simulink model "Chapter_9_Section_3_3"  (R2026a)
settings: Solver=FixedStepAuto  FixedStep=0.02  EnableMultiTasking=on
libraries: arduinolib x2, simulink x1
settings Model: SILPILModeSetting=veronly  ExtModeTrigDuration=2  Creator=ASUS  LastModifiedBy=ASUS
settings HardwareCC: ProdBitPerInt=16.0  ProdBitPerPointer=16.0  ProdBitPerSizeT=16.0  ProdBitPerPtrDiffT=16.0  ProdWordSize=8.0  ProdHWDeviceType=Atmel->AVR  UseEmbeddedCoderFeatures=off
settings RTWCC: SystemTargetFile=ert.tlc  HardwareBoard=Arduino Mega 2560  TLCOptions=-aInlineSetEventsForThisBaseRateFcn=TLC_FALSE -aSuppressMultiTaskScheduler=TLC_FALSE -aRateBasedStepFcn=1  Toolchain=Arduino AVR  BuildConfiguration=Faster Runs  Description=Embedded Coder
settings ERTTargetCC: ExtModeTransport=3.0  ExtModeAutomaticAllocSize=off  ExtModeStaticAllocSize=2048.0  SupportContinuousTime=on  SupportNonInlinedSFcns=on  SupportVariableSizeSignals=on

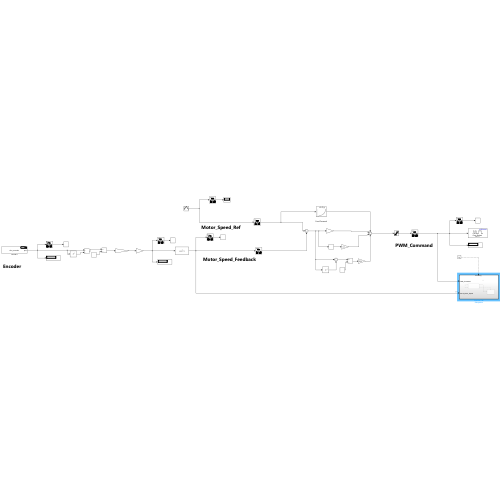
[thumbnail: Simulink's stored preview of the top-level diagram]
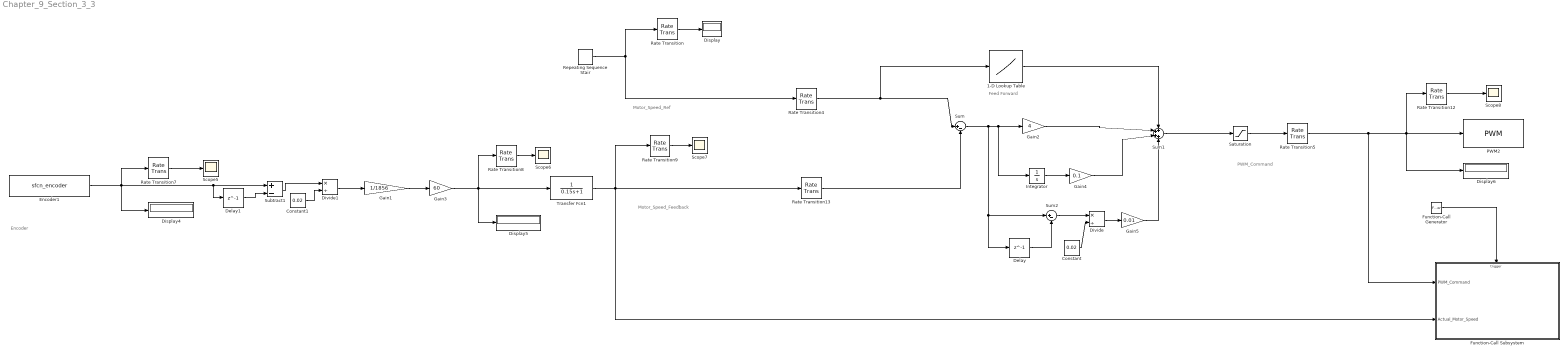
== system Chapter_9_Section_3_3 ==
  note: Feed Forward
  note: Motor_Speed_Ref
  note: Motor_Speed_Feedback
  note: PWM_Command
  note: Encoder
  1-D Lookup Table : Lookup_n-D  NumberOfTableDimensions=1  BreakpointsForDimension1=[78.1 185.9 260.2 305.1 331.5 351 363.3 374.1 382.7 394.4]  Table=[25.5 50.1 76.5 102 127.5 153 178.5 204 229.5 255]  InternalRulePriority=Speed  RndMeth=Simplest
  Constant : Constant  Value=0.02
  Constant1 : Constant  Value=0.02
  Delay : Delay  DelayLength=1  InitialCondition=0
  Delay1 : Delay  DelayLength=1  InitialCondition=0
  Display{,4..6} (4 alike) : Display
  Divide : Product  Inputs=*/
  Divide1 : Product  Inputs=*/
  Encoder1 : S-Function  InitFcn=try, set_param(gcb,'FunctionName','sfcn_encoder'), end  FunctionName=sfcn_encoder  Parameters=uint8(0),uint8(2),uint8(3)  SFunctionModules=sfcn_encoder_wrapper.c  SFunctionDeploymentMode=off  EnableBusSupport=off  mask(S-Function Builder){}
      mask init:
      | val = [[.9  0.75 0.75 1 1 .9 .9 1]',[1 1 0.75 0.75 .9 .9 1 .9]'];try , sys = get_param(gcb,'SfunBuilderFcnName');if isempty(sys), sys = get_param(gcb,'FunctionName'); end,catch, sys = get_param(gcb,'FunctionName'); end
      settings: CopyFcn=set_param(gcbh,'LinkStatus','none')  PreSaveFcn=try, set_param(gcb,'FunctionName','sfcn_encoder'), end  OpenFcn=sfunctionwizard(gcbh)
      mask Display:
      | plot(val(:,1),val(:,2))
      | disp(sys)
      | port_label('output',1,sprintf('%s', 'pos'),'interpreter','tex')
  Function-Call Generator : FunctionCallGenerator  SampleTime=0.1
  Function-Call Subsystem : Subsystem  TreatAsAtomicUnit=on
  Gain1 : Gain  Gain=1/1856
  Gain2 : Gain  Gain=4
  Gain3 : Gain  Gain=60
  Gain4 : Gain  Gain=0.1
  Gain5 : Gain  Gain=0.01
  Integrator : Integrator
  PWM2 : arduinolib/PWM  pinNumber=5  frequencyType=Default  desiredFrequency=490.2  achievableFrequency=490.1961
  Rate Transition{,4..5,7..9,12..13} (8 alike) : RateTransition
  Repeating Sequence Stair : simulink/Sources/Repeating Sequence Stair  OutValues=[110:200 199:-1:110]  tsamp=0.2  OutMin=[]  OutMax=[]  OutDataTypeStr=double  OutputDataTypeScalingMode=double  OutDataType=fixdt(0,8)  ConRadixGroup=Best Precision: Vector-wise  OutScaling=2^-12
  Saturation : Saturate  UpperLimit=255  LowerLimit=0
  Scope{5..8} (4 alike) : Scope
      Scope5 settings: ActiveDisplayYMinimum=-22.407200582277603  ActiveDisplayYMaximum=19.171363005949797  DataLoggingVariableName=ScopeData5
      Scope6 settings: ActiveDisplayYMinimum=-22.407200582277603  ActiveDisplayYMaximum=19.171363005949797  DataLoggingVariableName=ScopeData6
      Scope7 settings: ActiveDisplayYMinimum=-22.407200582277603  ActiveDisplayYMaximum=19.171363005949797  DataLoggingVariableName=ScopeData7
      Scope8 settings: ActiveDisplayYMinimum=-11.899191623313698  ActiveDisplayYMaximum=179.03299178469436  DataLoggingVariableName=ScopeData8
  Subtract1 : Sum  Inputs=+-
  Sum : Sum  Inputs=|+-
  Sum1 : Sum  Inputs=++++
  Sum2 : Sum  Inputs=|+-
  Transfer Fcn1 : TransferFcn  Denominator=[0.15 1]
  wires:
  Gain4/1 -> Sum1/3
  Divide/1 -> Gain5/1
  Gain5/1 -> Sum1/4
  Delay/1 -> Sum2/2
  Constant/1 -> Divide/2
  Sum1/1 -> Saturation/1
  Sum2/1 -> Divide/1
  Integrator/1 -> Gain4/1
  1-D Lookup Table/1 -> Sum1/1
  Rate Transition13/1 -> Sum/2
  Rate Transition4/1 -> 1-D Lookup Table/1, Sum/1
  Gain2/1 -> Sum1/2
  Sum/1 -> Sum2/1, Delay/1, Integrator/1, Gain2/1
  Saturation/1 -> Rate Transition5/1
  Rate Transition8/1 -> Scope6/1
  Delay1/1 -> Subtract1/2
  Rate Transition7/1 -> Scope5/1
  Subtract1/1 -> Divide1/1
  Transfer Fcn1/1 -> Function-Call Subsystem/2(Actual_Motor_Speed), Rate Transition13/1, Rate Transition9/1
  Rate Transition9/1 -> Scope7/1
  Gain1/1 -> Gain3/1
  Divide1/1 -> Gain1/1
  Constant1/1 -> Divide1/2
  Encoder1/1 -> Subtract1/1, Delay1/1, Rate Transition7/1, Display4/1
  Gain3/1 -> Transfer Fcn1/1, Display5/1, Rate Transition8/1
  Repeating Sequence Stair/1 -> Rate Transition4/1, Rate Transition/1
  Rate Transition/1 -> Display/1
  Rate Transition12/1 -> Scope8/1
  Rate Transition5/1 -> Function-Call Subsystem/1(PWM_Command), Display6/1, Rate Transition12/1, PWM2/1
  Function-Call Generator/1 -> Function-Call Subsystem/Trigger

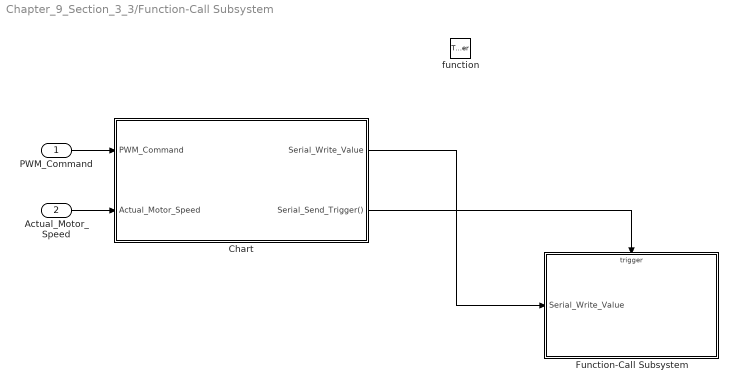
== system Chapter_9_Section_3_3/Function-Call Subsystem ==
  PWM_Command : Inport
  Actual_Motor_Speed : Inport  Port=2
  function : TriggerPort  TriggerType=function-call  VariantControl=(inherit)
  Chart : Stateflow chart  TreatAsAtomicUnit=on
  Function-Call Subsystem : Subsystem  TreatAsAtomicUnit=on
  wires:
  PWM_Command/1 -> Chart/1(PWM_Command)
  Actual_Motor_Speed/1 -> Chart/2(Actual_Motor_Speed)
  Chart/1(Serial_Write_Value) -> Function-Call Subsystem/1(Serial_Write_Value)
  Chart/2(Serial_Send_Trigger()) -> Function-Call Subsystem/Trigger

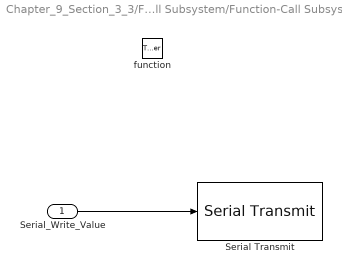
== system Chapter_9_Section_3_3/Function-Call Subsystem/Function-Call Subsystem ==
  Serial_Write_Value : Inport
  function : TriggerPort  TriggerType=function-call  VariantControl=(inherit)
  Serial Transmit : arduinolib/Serial Transmit  portNumber=1  sendmode=println  sendformat=Decimal  floatprecision=2  header=[]  terminator=[]  blockPlatform=ARDUINO
  wires:
  Serial_Write_Value/1 -> Serial Transmit/1

== stateflow chart Chapter_9_Section_3_3/Function-Call Subsystem/Chart ==
  (default) -> (junction 5) : {Serial_Write_Value = PWM_Command;
      | Serial_Send_Trigger;
      | Serial_Write_Value = Actual_Motor_Speed;
      | Serial_Send_Trigger;}
  data: PWM_Command input; Actual_Motor_Speed input; Serial_Write_Value output
  events: Serial_Send_Trigger output FUNCTION_CALL_EVENT
